simulink library "ddm"  (R2021b)
settings: Solver=VariableStepAuto  StartTime=0.0  StopTime=10.0  RelTol=1e-3
undefined symbols (not defined in the file or in its folder): ENUM_ADASACCSTA_ERROR, ENUM_ADASACCSTA_OFF, ENUM_ADASACCSTA_STANDBY, ENUM_ADASISASTA_OFF, ENUM_ALLOWMOV_ALLOWREADY, ENUM_APS, ENUM_BRKSTA_ERROR, ENUM_BRKSTA_OFF, ENUM_BRKSTA_ON, ENUM_BRKSW_INVALID, ENUM_BRKSW_OFF, ENUM_BRKSW_ON, ENUM_CHGPREACTERRSTA_OBCPRE, ENUM_DCDCFAULTSTA_ANYFAULTLV1, ENUM_DCDCFAULTSTA_ANYFAULTLV2, ENUM_DRIVETRAIN_AWD, ENUM_DRIVETRAIN_FWD, ENUM_DRIVETRAIN_RWD, ENUM_DRSEATSTA_INVALID, ENUM_EDUDRTSTA_NORMAL, ENUM_EPBSTA_APPLIED, ENUM_EPBSTA_RELEASED, ENUM_HVBATTREADYPRE_READY, ENUM_MCUWARN_LV0, ENUM_MCUWARN_LV1, ENUM_MCUWARN_LV2, ENUM_MCUWARN_LV3, ENUM_MCUWARN_NOERROR, ENUM_OBCFAULTSTA_ANYFAULT, ENUM_PAS_R2F2, ENUM_PDFAULT_BATTPDFAIL, ENUM_PDFAULT_DCDCDISABLE, ENUM_PDFAULT_MCUDISABLE, ENUM_PDFAULT_MCUDISCHRG, ENUM_POWERSTA_OFF, ENUM_POWERSTA_ON, ENUM_POWERSTA_READY, ENUM_POWERSTA_STANDBY, ENUM_PRESSINDI_LOW, ENUM_PUFAULT_BATTUPFAIL, ENUM_PUFAULT_DCDCENABLEFAIL, ENUM_PUFAULT_PRECHRGCHKFAIL, ENUM_PUFAULT_SAFETYCHKFAIL, ENUM_PUSTATE_COMPLETED, ENUM_PWRSTASW_OFF, ENUM_PWRSTASW_OFFA, ENUM_PWRSTASW_OFFCHVCHRG, ENUM_PWRSTASW_OFFCLVCHRG, ENUM_PWRSTASW_ON, ENUM_PWRSTASW_ONHVCHRG, ENUM_PWRSTASW_READY, ENUM_PWRSTASW_STANDBY, ENUM_RANGESTA_12IN, ENUM_SHIFTCOMMAND_D, ENUM_SHIFTCOMMAND_N, ENUM_SHIFTCOMMAND_P, ENUM_SHIFTCOMMAND_R, ENUM_VEHMALFUNLV_2ND, ENUM_VEHMALFUNLV_3RD, ENUM_VEHMALFUNLV_4TH ... (+835)
libraries: hcu_lib x750, $bdroot x12, simulink x5
(part 15 of 28)

== system ddm/DDM/DDM/PMM/Brake switch signal abnormal/Brake switch signal abnormal and no backup signal ==
  note: Diagnostics and Fault Handling
  note: Release Condition During Failure Detection
  note: Test Detection Criteria
  note: Release Condition After Failure Decision
  note: Fail Safe Operation During Failure Detection
  note: Test Pass Criteria
  note: Fail Safe Operation After Failure Decision
  task_time_s : Inport
  VPMM_PowerSta_enum : Inport  Port=2
  VPMM_PwrStaSW_enum : Inport  Port=3
  BrkSWNoBac : Inport  Port=4
  BrkSWPass : Inport  Port=5
  DTC_clear_request : Inport  Port=6
  VDDM_BrakeSW_enum : Inport  Port=7
  Constant1 : Constant  Value=ENUM_PWRSTASW_READY
  Constant11 : Constant  Value=KDDM_BrkSWNoBacPassSW_flg
  Constant15 : Constant  Value=KDDM_BrkSWNoBacCFSSW_flg
  Constant19 : Constant  Value=ENUM_POWERSTA_OFF
  Constant2 : Constant  Value=ENUM_PWRSTASW_ON
  Constant20 : Constant  Value=KDDM_BrkSWNoBacDFSSW_flg
  Constant23 : Constant  Value=TRUE
  Constant24 : Constant  Value=TRUE
  Constant25 : Constant  Value=FALSE
  Constant26 : Constant  Value=ENUM_PWRSTASW_READY
  Constant27 : Constant  Value=FALSE
  Constant28 : Constant  Value=ENUM_PWRSTASW_ON
  Constant29 : Constant  Value=ENUM_PWRSTASW_ONHVCHRG
  Constant3 : Constant  Value=ENUM_PWRSTASW_ONHVCHRG
  Constant38 : Constant  Value=KDDM_BrkSWNoBacDetTO_s
  Constant4 : Constant  Value=KDDM_BrkSWNoBacPassTO_s
  Constant40 : Constant  Value=KDDM_BrkSWNoBacDTC_cnt
  Constant42 : Constant  Value=ENUM_DRSEATSTA_INVALID
  Constant43 : Constant  Value=KDDM_BrkSWNoBacPassTO_s
  Constant44 : Constant  Value=KDDM_BrkSWNoBacDetSW_flg
  Constant5 : Constant  Value=KDDM_BrkSWNoBacDTC_cnt
  Constant8 : Constant  Value=FALSE
  DTC_Couter : hcu_lib/Basic_Blocks/DTC_Couter
  DTC_Info : hcu_lib/Basic_Blocks/DTC_Info
  Data Type Conversion1 : DataTypeConversion  OutDataTypeStr=uint8
  Equal{1..2,4..8} (7 alike) : RelationalOperator  Operator===  OutDataTypeStr=boolean  RndMeth=Simplest
  Equal3 : RelationalOperator  OutDataTypeStr=boolean  RndMeth=Simplest
  Logical Operator1 : Logic  Operator=NOT  AllPortsSameDT=off  OutDataTypeStr=boolean
  Logical Operator12 : Logic  AllPortsSameDT=off  OutDataTypeStr=boolean
  Logical Operator15 : Logic  AllPortsSameDT=off  OutDataTypeStr=boolean
  Logical Operator18 : Logic  AllPortsSameDT=off  OutDataTypeStr=boolean
  Logical Operator19 : Logic  Inputs=3  AllPortsSameDT=off  OutDataTypeStr=boolean
  Logical Operator2 : Logic  Operator=OR  Inputs=3  AllPortsSameDT=off  OutDataTypeStr=boolean
  Logical Operator3 : Logic  Operator=OR  Inputs=3  AllPortsSameDT=off  OutDataTypeStr=boolean
  Logical Operator4 : Logic  Operator=OR  AllPortsSameDT=off  OutDataTypeStr=boolean
  Logical Operator5 : Logic  Operator=OR  Inputs=3  AllPortsSameDT=off  OutDataTypeStr=boolean
  Logical Operator6 : Logic  Operator=NOT  AllPortsSameDT=off  OutDataTypeStr=boolean
  Logical Operator7 : Logic  Operator=OR  AllPortsSameDT=off  OutDataTypeStr=boolean
  Logical Operator8 : Logic  Operator=OR  AllPortsSameDT=off  OutDataTypeStr=boolean
  Relay : Relay  OnSwitchValue=ONE_INT  OffSwitchValue=ZERO_INT
  SR_Latch1 : Subsystem  mask(SR_Latch){}
      mask help: SR latch function.
  SR_Latch3 : hcu_lib/Basic_Blocks/SR_Latch
  SR_Latch4 : hcu_lib/Basic_Blocks/SR_Latch
  Switch{,2,4..6} (5 alike) : Switch  Criteria=u2 ~= 0
  Test Detection Criteria : hcu_lib/Basic_Blocks/Test Detection Criteria
  Timer1 : hcu_lib/Basic_Blocks/Timer
  VDDM_BrkSWNoBacDTC_raw32 : Outport
  VDDM_VCUBrkSWSta_enum : Outport  Port=2
  wires:
  Relay/1 -> SR_Latch3/1
  Data Type Conversion1/1 -> [VDDM_BrkSWNoBacDTC_cnt]  "VDDM_BrkSWNoBacDTC_cnt"
  Logical Operator19/1 -> DTC_Couter/1
  DTC_Couter/1 -> SR_Latch4/1
  Constant15/1 -> Logical Operator18/2
  [VDDM_BrkSWNoBacCFS_flg] -> Logical Operator7/1
  Constant44/1 -> Logical Operator19/2
  Logical Operator4/1 -> SR_Latch4/2
  SR_Latch3/1 -> Logical Operator12/2
  [VDDM_BrkSWNoBacCFSRls_flg] -> Logical Operator3/2
  [DTC_clear_request] -> Logical Operator1/1
  Logical Operator1/1 -> Logical Operator19/3
  [VDDM_BrkSWNoBacDTC_cnt] -> Relay/1
  DTC_Couter/2 -> Data Type Conversion1/1
  Logical Operator18/1 -> [VDDM_BrkSWNoBacCFS_flg]  "VDDM_BrkSWNoBacCFS_flg"
  Constant11/1 -> Logical Operator15/2
  [VDDM_BrkSWNoBacDet_flg] -> Logical Operator19/1
  Constant20/1 -> Logical Operator12/1
  Logical Operator7/1 -> SR_Latch3/2
  [VDDM_BrkSWNoBacPass_flg] -> Logical Operator3/1
  Constant5/1 -> DTC_Couter/3
  SR_Latch4/1 -> Logical Operator18/1
  Logical Operator3/1 -> Logical Operator15/1
  [VDDM_BrkSWNoBacCFSRls_flg] -> Logical Operator4/1
  Logical Operator12/1 -> [VDDM_BrkSWNoBacDFS_flg]  "VDDM_BrkSWNoBacDFS_flg"
  Logical Operator15/1 -> DTC_Couter/2
  [DTC_clear_request] -> Logical Operator4/2
  [DTC_clear_request] -> Logical Operator7/2
  [DTC_clear_request] -> Logical Operator3/3
  VDDM_BrakeSW_enum/1 -> [VDDM_BrakeSW_enum]
  Constant8/1 -> Switch6/1
  Switch5/1 -> Switch6/3
  Switch6/1 -> Test Detection Criteria/1
  [DTC_clear_request] -> Switch6/2
  [DTC_clear_request] -> DTC_Info/4
  Constant38/1 -> Test Detection Criteria/4
  [VDDM_BrkSWNoBacDet_flg] -> DTC_Info/1
  BrkSWPass/1 -> Switch2/1
  BrkSWNoBac/1 -> Switch5/1
  [VDDM_BrkSWNoBacCFS_flg] -> DTC_Info/3
  [VDDM_BrkSWNoBacPass_flg] -> DTC_Info/2
  DTC_Info/1 -> VDDM_BrkSWNoBacDTC_raw32/1  "VDDM_BrkSWNoBacDTC_raw32"
  [task_time_s] -> Timer1/3
  DTC_clear_request/1 -> [DTC_clear_request]
  [VDDM_VCUBrkSWSta_enum] -> VDDM_VCUBrkSWSta_enum/1
  Constant26/1 -> Equal1/2
  [VPMM_PwrStaSW_enum] -> Equal1/1
  Constant40/1 -> Test Detection Criteria/3
  [VPMM_PwrStaSW_enum] -> Equal5/1
  [VPMM_PwrStaSW_enum] -> Equal6/1
  Logical Operator2/1 -> Switch5/2
  Switch/1 -> [VDDM_VCUBrkSWSta_enum]  "VDDM_VCUBrkSWSta_enum"
  SR_Latch1/1(latched) -> [VDDM_BrkSWNoBacPass_flg]  "VDDM_BrkSWNoBacPass_flg"
  [VPMM_PowerSta_enum] -> Equal4/1
  Constant24/1 -> Switch4/1
  Constant42/1 -> Switch/1
  Switch2/1 -> Timer1/1, Logical Operator6/1, SR_Latch1/2(reset)
  Equal3/1 -> SR_Latch1/1(set)
  Switch4/1 -> [VDDM_BrkSWNoBacCFSRls_flg]  "VDDM_BrkSWNoBacCFSRls_flg"
  Constant19/1 -> Equal4/2
  Constant25/1 -> Switch4/3
  [DTC_clear_request] -> Logical Operator8/2
  Logical Operator8/1 -> Switch4/2
  Equal4/1 -> Logical Operator8/1
  Constant27/1 -> Switch5/3
  Constant23/1 -> Switch2/3
  [VDDM_BrkSWNoBacCFS_flg] -> Switch/2
  [VDDM_BrakeSW_enum] -> Switch/3
  Test Detection Criteria/1 -> [VDDM_BrkSWNoBacDet_flg]  "VDDM_BrkSWNoBacDet_flg"
  [task_time_s] -> Test Detection Criteria/2
  Timer1/1 -> Equal3/1
  Constant43/1 -> Timer1/4
  Constant29/1 -> Equal6/2
  Constant4/1 -> Equal3/2
  Constant28/1 -> Equal5/2
  VPMM_PowerSta_enum/1 -> [VPMM_PowerSta_enum]
  VPMM_PwrStaSW_enum/1 -> [VPMM_PwrStaSW_enum]
  task_time_s/1 -> [task_time_s]
  Logical Operator6/1 -> Timer1/2
  Equal5/1 -> Logical Operator2/1
  Equal1/1 -> Logical Operator2/2
  Equal6/1 -> Logical Operator2/3
  [VPMM_PwrStaSW_enum] -> Equal2/1
  Constant2/1 -> Equal7/2
  [VPMM_PwrStaSW_enum] -> Equal8/1
  Equal2/1 -> Logical Operator5/2
  Equal7/1 -> Logical Operator5/1
  Equal8/1 -> Logical Operator5/3
  Logical Operator5/1 -> Switch2/2
  [VPMM_PwrStaSW_enum] -> Equal7/1
  Constant3/1 -> Equal8/2
  Constant1/1 -> Equal2/2

== system ddm/DDM/DDM/PMM/Brake switch signal abnormal/Subsystem ==
  note: 17
  note: 6
  note: 35
  note: 25
  note: 27
  note: 30
  note: 12
  note: 19
  note: 3
  note: 21
  note: 1
  note: 9
  note: 11
  note: 36
  note: 24
  note: 33
  note: 29
  note: 13
  note: 5
  note: 23
  note: 18
  note: 15
  VDDM_CANBSW2S_enum : Inport
  BrakeSW : Inport  Port=2
  Brake_Stop_Lamp : Inport  Port=3
  BrkPedalPos_enum : Inport  Port=4
  1-D Lookup Table : Lookup_n-D  NumberOfTableDimensions=1  BreakpointsForDimension1=[1:36]  Table=[20,8,32,18,6,30,19,7,31,16,4,28,17,5,29,15,3,27,14,2,26,13,1,25,24,12,36,23,11,35,22,10,34,21,9,33]  ExtrapMethod=Clip  InternalRulePriority=Speed  RndMeth=Simplest  InputSameDT=on
  AND{,2..7,10,12..25} (22 alike) : Logic  Inputs=4  AllPortsSameDT=off  OutDataTypeStr=boolean
  AND1 : Logic  Operator=OR  Inputs=6  AllPortsSameDT=off  OutDataTypeStr=boolean
  AND11 : Logic  Operator=OR  Inputs=15  AllPortsSameDT=off  OutDataTypeStr=boolean
  AND8 : Logic  Operator=OR  AllPortsSameDT=off  OutDataTypeStr=boolean
  AND9 : Logic  Operator=OR  AllPortsSameDT=off  OutDataTypeStr=boolean
  Constant{1..10,15,17..18,23,29..30,32} (17 alike) : Constant  Value=ENUM_BRKSTA_ON
  Constant11 : Constant  Value=ENUM_BRKSW_OFF
  Constant{16,19,21,25..28,31,38,50,53,55,57,59..61} (16 alike) : Constant  Value=ENUM_BRKSTA_ERROR
  Constant{20,22,24,33..34,39,41..44} (10 alike) : Constant  Value=ENUM_BRKSTA_OFF
  Constant35 : Constant  Value=FALSE
  Constant36 : Constant  Value=TRUE
  Constant37 : Constant  Value=0
  Constant40 : Constant  Value=0
  Constant46 : Constant  Value=ENUM_BRKSW_ON
  Constant47 : Constant  Value=ENUM_BRKSW_INVALID
  Data Type Conversion{,1..3} (4 alike) : DataTypeConversion
  Equal{1..45} (45 alike) : RelationalOperator  Operator===  OutDataTypeStr=boolean  RndMeth=Simplest
  OR{,1..21} (22 alike) : Logic  Operator=NOT  AllPortsSameDT=off  OutDataTypeStr=boolean
  Switch6 : Switch  Criteria=u2 > Threshold
  Switch7 : Switch  Criteria=u2 > Threshold
  Switch8 : Switch  Criteria=u2 > Threshold
  n-D Lookup Table : Lookup_n-D  NumberOfTableDimensions=4  BreakpointsForDimension1=[0:2]  BreakpointsForDimension2=[0:1]  BreakpointsForDimension3=[0:1]  BreakpointsForDimension4=[0:2]  Table=reshape(1:36,[3,2,2,3])  ExtrapMethod=Clip  InternalRulePriority=Speed  RndMeth=Simplest  InputSameDT=on
      settings: InputPortMap=u0,u1,u2,u3
  BrkSWErr : Outport
  BrkSWNoBac : Outport  Port=2
  BrkSWPass : Outport  Port=3
  VDDM_BrakeSW_enum : Outport  Port=4
  wires:
  [VDDM_BrakeSW_enum] -> VDDM_BrakeSW_enum/1
  [BrkSWPass] -> BrkSWPass/1
  [BrkSWNoBac] -> BrkSWNoBac/1
  [BrkSWErr] -> BrkSWErr/1
  BrkPedalPos_enum/1 -> [BrkPedalPos_enum]
  Brake_Stop_Lamp/1 -> [Brake_Stop_Lamp]
  BrakeSW/1 -> [BrakeSW]
  VDDM_CANBSW2S_enum/1 -> [VDDM_CANBSW2S_enum]
  AND4/1 -> AND1/4
  Constant28/1 -> Equal14/2
  AND25/1 -> AND11/15
  Constant31/1 -> Equal13/2
  Equal22/1 -> AND10/3
  Constant7/1 -> Equal3/2
  Equal33/1 -> AND19/4
  Equal39/1 -> AND22/4
  OR1/1 -> AND2/3
  [Brake_Stop_Lamp] -> OR8/1
  [Brake_Stop_Lamp] -> OR10/1
  Constant8/1 -> Equal8/2
  Equal17/1 -> AND7/1
  Constant50/1 -> Equal35/2
  Constant32/1 -> Equal41/2
  [BrkPedalPos_enum] -> Equal35/1
  Equal43/1 -> AND24/4
  Constant33/1 -> Equal26/2
  [VDDM_CANBSW2S_enum] -> Equal9/1
  Constant37/1 -> Equal20/2
  [BrkPedalPos_enum] -> Equal45/1
  Switch7/1 -> Switch8/3
  Equal36/1 -> AND21/1
  [Brake_Stop_Lamp] -> AND5/3
  Constant3/1 -> Equal17/2
  Constant44/1 -> Equal43/2
  Constant39/1 -> Equal30/2
  OR8/1 -> AND13/3
  [Brake_Stop_Lamp] -> OR19/1
  [VDDM_CANBSW2S_enum] -> Equal20/1
  Equal20/1 -> AND10/1
  [Brake_Stop_Lamp] -> Equal22/1
  [BrkPedalPos_enum] -> Equal6/1
  [VDDM_CANBSW2S_enum] -> Equal2/1
  Equal5/1 -> AND3/1
  [Brake_Stop_Lamp] -> OR3/1
  [Brake_Stop_Lamp] -> OR15/1
  Constant26/1 -> Equal11/2
  [Brake_Stop_Lamp] -> AND21/3
  OR19/1 -> AND24/3
  [BrkPedalPos_enum] -> Equal10/1
  [BrakeSW] -> AND25/2
  OR3/1 -> AND4/3
  Equal31/1 -> AND18/4
  [BrkPedalPos_enum] -> Equal31/1
  [VDDM_CANBSW2S_enum] -> Equal38/1
  Equal13/1 -> AND6/4
  AND9/1 -> Switch6/2
  [VDDM_CANBSW2S_enum] -> Equal17/1
  AND14/1 -> AND11/4
  [Brake_Stop_Lamp] -> AND16/3
  Equal18/1 -> AND7/4
  [BrkPedalPos_enum] -> Equal27/1
  Constant61/1 -> Equal44/2
  Equal14/1 -> AND6/1
  [VDDM_CANBSW2S_enum] -> Equal5/1
  [VDDM_CANBSW2S_enum] -> Equal28/1
  [VDDM_CANBSW2S_enum] -> Equal3/1
  [BrkPedalPos_enum] -> Equal8/1
  [Brake_Stop_Lamp] -> OR14/1
  AND17/1 -> AND11/7
  Constant30/1 -> Equal16/2
  Constant43/1 -> Equal34/2
  OR13/1 -> AND18/2
  Equal26/1 -> AND16/1
  OR7/1 -> AND13/2
  [BrakeSW] -> AND24/2
  Equal16/1 -> AND/1
  Equal34/1 -> AND20/1
  Equal9/1 -> AND14/1
  Equal12/1 -> AND5/4
  [VDDM_CANBSW2S_enum] -> Equal24/1
  Constant16/1 -> Equal1/2
  Constant18/1 -> Equal31/2
  Constant9/1 -> Equal9/2
  AND2/1 -> AND1/2
  Constant40/1 -> Equal19/2
  OR17/1 -> AND23/2
  AND5/1 -> AND1/5
  AND6/1 -> AND1/6
  Equal37/1 -> AND21/4
  Constant25/1 -> Equal10/2
  [BrkPedalPos_enum] -> Equal15/1
  Constant21/1 -> Equal6/2
  [BrkPedalPos_enum] -> Equal29/1
  [VDDM_CANBSW2S_enum] -> Equal34/1
  [BrkPedalPos_enum] -> Equal23/1
  AND19/1 -> AND11/9
  Constant15/1 -> Equal27/2
  Equal27/1 -> AND16/4
  OR14/1 -> AND19/3
  [BrkPedalPos_enum] -> Equal43/1
  [VDDM_CANBSW2S_enum] -> Equal26/1
  [BrakeSW] -> AND16/2
  AND15/1 -> AND11/5
  Equal24/1 -> AND2/1
  Constant6/1 -> Equal23/2
  AND10/1 -> AND8/1
  OR11/1 -> AND17/3
  [BrakeSW] -> AND14/2
  [BrakeSW] -> AND17/2
  Constant38/1 -> Equal21/2
  [BrkPedalPos_enum] -> Equal41/1
  [BrakeSW] -> AND3/2
  Equal7/1 -> AND4/1
  Equal28/1 -> AND17/1
  OR16/1 -> AND22/3
  AND13/1 -> AND11/3
  Equal23/1 -> AND12/4
  Equal25/1 -> AND15/1
  Constant57/1 -> Equal40/2
  [VDDM_CANBSW2S_enum] -> Equal11/1
  Constant55/1 -> Equal38/2
  OR6/1 -> AND10/2
  AND16/1 -> AND11/6
  Equal10/1 -> AND4/4
  OR9/1 -> AND14/3
  AND8/1 -> AND9/2, [BrkSWPass]
  Constant1/1 -> Equal24/2
  [BrakeSW] -> AND20/2
  Equal19/1 -> AND10/4
  Constant36/1 -> Switch6/3
  [VDDM_CANBSW2S_enum] -> Equal40/1
  [BrakeSW] -> AND19/2
  [BrkPedalPos_enum] -> Equal1/1
  AND12/1 -> AND11/2
  Constant4/1 -> Equal18/2
  [VDDM_CANBSW2S_enum] -> Equal14/1
  [Brake_Stop_Lamp] -> AND/3
  [BrkPedalPos_enum] -> Equal37/1
  Constant60/1 -> Equal45/2
  Constant5/1 -> Equal2/2
  Constant20/1 -> Equal5/2
  [BrakeSW] -> AND22/2
  [BrakeSW] -> AND21/2
  Constant53/1 -> Equal36/2
  Equal35/1 -> AND20/4
  [VDDM_CANBSW2S_enum] -> Equal16/1
  [BrakeSW] -> OR7/1
  Constant10/1 -> Equal25/2
  [Brake_Stop_Lamp] -> OR5/1
  [Brake_Stop_Lamp] -> AND3/3
  Equal6/1 -> AND3/4
  Constant42/1 -> Equal33/2
  AND22/1 -> AND11/12
  AND7/1 -> AND8/2, AND11/1
  [VDDM_CANBSW2S_enum] -> Equal30/1
  [BrakeSW] -> OR/1
  Equal41/1 -> AND23/4
  OR12/1 -> AND18/3
  [Brake_Stop_Lamp] -> OR12/1
  [VDDM_CANBSW2S_enum] -> Equal36/1
  Constant24/1 -> Equal15/2
  [Brake_Stop_Lamp] -> OR16/1
  Constant41/1 -> Equal32/2
  Equal32/1 -> AND19/1
  Switch8/1 -> [VDDM_BrakeSW_enum]
  Constant17/1 -> Equal29/2
  Equal45/1 -> AND25/4
  Constant19/1 -> Equal4/2
  [BrakeSW] -> AND7/2
  OR21/1 -> AND7/3
  Constant47/1 -> Switch8/1
  [Brake_Stop_Lamp] -> OR21/1
  [Brake_Stop_Lamp] -> OR9/1
  Equal40/1 -> AND23/1
  Equal3/1 -> AND13/1
  Equal11/1 -> AND5/1
  Equal38/1 -> AND22/1
  Constant11/1 -> Switch7/3
  Equal1/1 -> AND/4
  Switch6/1 -> [BrkSWErr]
  [BrkPedalPos_enum] -> Equal13/1
  [BrkPedalPos_enum] -> Equal21/1
  AND24/1 -> AND11/14
  Constant35/1 -> Switch6/1
  AND/1 -> AND1/1
  Constant34/1 -> Equal28/2
  [VDDM_CANBSW2S_enum] -> Equal44/1
  OR10/1 -> AND15/3
  [Brake_Stop_Lamp] -> AND12/3
  [BrkPedalPos_enum] -> Equal18/1
  Equal8/1 -> AND13/4
  Equal2/1 -> AND12/1
  [BrkPedalPos_enum] -> Equal4/1
  [Brake_Stop_Lamp] -> OR11/1
  Equal44/1 -> AND25/1
  Equal42/1 -> AND24/1
  [BrakeSW] -> OR4/1
  OR20/1 -> AND25/3
  [VDDM_CANBSW2S_enum] -> Equal7/1
  OR4/1 -> AND6/2
  Constant23/1 -> Equal37/2
  [VDDM_CANBSW2S_enum] -> Equal32/1
  [VDDM_CANBSW2S_enum] -> Equal42/1
  [BrkPedalPos_enum] -> Equal19/1
  [BrkPedalPos_enum] -> Equal12/1
  AND21/1 -> AND11/11
  [BrkPedalPos_enum] -> Equal39/1
  [BrakeSW] -> OR6/1
  Constant59/1 -> Equal42/2
  AND1/1 -> [BrkSWNoBac], AND9/1, Switch8/2
  AND23/1 -> AND11/13
  Constant27/1 -> Equal12/2
  AND18/1 -> AND11/8
  AND20/1 -> AND11/10
  [BrakeSW] -> AND15/2
  Constant46/1 -> Switch7/1
  AND11/1 -> Switch7/2
  [BrakeSW] -> OR2/1
  [VDDM_CANBSW2S_enum] -> Equal25/1
  Constant2/1 -> Equal22/2
  [Brake_Stop_Lamp] -> OR1/1
  [Brake_Stop_Lamp] -> OR18/1
  [BrakeSW] -> OR13/1
  OR5/1 -> AND6/3
  Constant22/1 -> Equal7/2
  Constant29/1 -> Equal39/2
  OR18/1 -> AND23/3
  [BrakeSW] -> AND/2
  [BrakeSW] -> OR17/1
  AND3/1 -> AND1/3
  [BrakeSW] -> AND12/2
  [Brake_Stop_Lamp] -> OR20/1
  OR15/1 -> AND20/3
  OR/1 -> AND2/2
  Equal21/1 -> AND15/4
  Equal30/1 -> AND18/1
  Equal29/1 -> AND17/4
  Equal15/1 -> AND14/4
  [BrakeSW] -> AND5/2
  OR2/1 -> AND4/2
  Equal4/1 -> AND2/4
  [BrkPedalPos_enum] -> Equal33/1
  Data Type Conversion2/1 -> n-D Lookup Table/3
  Data Type Conversion3/1 -> n-D Lookup Table/4
  Data Type Conversion1/1 -> n-D Lookup Table/2
  Data Type Conversion/1 -> n-D Lookup Table/1
  [BrakeSW] -> Data Type Conversion1/1
  [BrkPedalPos_enum] -> Data Type Conversion3/1
  n-D Lookup Table/1 -> 1-D Lookup Table/1
  [Brake_Stop_Lamp] -> Data Type Conversion2/1
  1-D Lookup Table/1 -> [VDDM_BrakeSigMatrix_enum]  "VDDM_BrakeSigMatrix_enum"
  [VDDM_CANBSW2S_enum] -> Data Type Conversion/1

== system ddm/DDM/DDM/PMM/Comm err/FDC lost communication with EPAS2 ==
  note: Diagnostics and Fault Handling
  note: Release Condition During Failure Detection
  note: Release Condition After Failure Decision
  note: Fail Safe During Detection
  note: Test Detection Criteria
  note: Test Pass Criteria
  note: Fail Safe After Decision
  task_time_s : Inport
  VPMM_PowerSta_enum : Inport  Port=2
  VPMM_PwrStaSW_enum : Inport  Port=3
  VDDM_C1EPAS2LCChk_flg : Inport  Port=4
  No_CAN1_BUS_OFF : Inport  Port=5
  DTC_clear_request : Inport  Port=6
  Constant15 : Constant  Value=KDDM_C1EPAS2LCCFSSW_flg
  Constant16 : Constant  Value=TRUE
  Constant18 : Constant  Value=KDDM_C1EPAS2LCPassTO_s
  Constant19 : Constant  Value=KDDM_C1EPAS2LCPassTO_s
  Constant{2,21,25,27} (4 alike) : Constant  Value=FALSE
  Constant20 : Constant  Value=KDDM_C1EPAS2LCDFSSW_flg
  Constant24 : Constant  Value=TRUE
  Constant26 : Constant  Value=ENUM_PWRSTASW_OFF
  Constant28 : Constant  Value=ENUM_PWRSTASW_OFF
  Constant3 : Constant  Value=TRUE
  Constant4 : Constant  Value=ENUM_POWERSTA_OFF
  Constant40 : Constant  Value=KDDM_C1EPAS2LCDTC_cnt
  Constant41 : Constant  Value=KDDM_C1EPAS2LCDetTO_s
  Constant46 : Constant  Value=KDDM_C1EPAS2LCDetSW_flg
  Constant48 : Constant  Value=KDDM_C1EPAS2LCDTC_cnt
  Constant5 : Constant  Value=KDDM_C1EPAS2LCPassSW_flg
  DTC_Couter : hcu_lib/Basic_Blocks/DTC_Couter
  DTC_Info : hcu_lib/Basic_Blocks/DTC_Info
  Data Type Conversion1 : DataTypeConversion  OutDataTypeStr=uint8
  Equal : RelationalOperator  Operator=~=  OutDataTypeStr=boolean  RndMeth=Simplest
  Equal2 : RelationalOperator  Operator=~=  OutDataTypeStr=boolean  RndMeth=Simplest
  Equal3 : RelationalOperator  OutDataTypeStr=boolean  RndMeth=Simplest
  Equal4 : RelationalOperator  Operator===  OutDataTypeStr=boolean  RndMeth=Simplest
  Goto19 : Goto  Commented=on  GotoTag=EDriveSysErr_VCUErr_flg
  Logical Operator1 : Logic  Operator=NOT  AllPortsSameDT=off  OutDataTypeStr=boolean
  Logical Operator{2,5,12,15,18} (5 alike) : Logic  AllPortsSameDT=off  OutDataTypeStr=boolean
  Logical Operator19 : Logic  Inputs=3  AllPortsSameDT=off  OutDataTypeStr=boolean
  Logical Operator3 : Logic  Operator=OR  Inputs=3  AllPortsSameDT=off  OutDataTypeStr=boolean
  Logical Operator4 : Logic  Operator=OR  AllPortsSameDT=off  OutDataTypeStr=boolean
  Logical Operator6 : Logic  Operator=NOT  AllPortsSameDT=off  OutDataTypeStr=boolean
  Logical Operator7 : Logic  Operator=OR  AllPortsSameDT=off  OutDataTypeStr=boolean
  Logical Operator8 : Logic  Operator=OR  AllPortsSameDT=off  OutDataTypeStr=boolean
  Relay : Relay  OnSwitchValue=ONE_INT  OffSwitchValue=ZERO_INT
  SR_Latch1 : Subsystem  mask(SR_Latch){}
      mask help: SR latch function.
  SR_Latch3 : hcu_lib/Basic_Blocks/SR_Latch
  SR_Latch4 : hcu_lib/Basic_Blocks/SR_Latch
  Switch{,1,4..6} (5 alike) : Switch  Criteria=u2 ~= 0
  Test Detection Criteria : hcu_lib/Basic_Blocks/Test Detection Criteria
  Timer1 : hcu_lib/Basic_Blocks/Timer
  VDDM_C1EPAS2LCDTC_raw32 : Outport
  VDDM_C1EPAS2LCCFS_flg : Outport  Port=2
  wires:
  [DTC_clear_request] -> Logical Operator1/1
  Logical Operator3/1 -> Logical Operator15/1
  Constant46/1 -> Logical Operator19/2
  SR_Latch4/1 -> Logical Operator18/1
  [DTC_clear_request] -> Logical Operator7/2
  [VDDM_C1EPAS2LCCFS_flg] -> Logical Operator7/1
  DTC_Couter/1 -> SR_Latch4/1
  Logical Operator7/1 -> SR_Latch3/2
  Logical Operator4/1 -> SR_Latch4/2
  Constant48/1 -> DTC_Couter/3
  [VDDM_C1EPAS2LCDet_flg] -> Logical Operator19/1
  SR_Latch3/1 -> Logical Operator12/2
  Logical Operator15/1 -> DTC_Couter/2
  Logical Operator19/1 -> DTC_Couter/1
  [VDDM_C1EPAS2LCDTC_cnt] -> Relay/1
  Constant20/1 -> Logical Operator12/1
  DTC_Couter/2 -> Data Type Conversion1/1
  [DTC_clear_request] -> Logical Operator3/3
  Logical Operator1/1 -> Logical Operator19/3
  [VDDM_C1EPAS2LCCFSRls_flg] -> Logical Operator4/1
  Relay/1 -> SR_Latch3/1
  [VDDM_C1EPAS2LCCFSRls_flg] -> Logical Operator3/2
  Data Type Conversion1/1 -> [VDDM_C1EPAS2LCDTC_cnt]  "VDDM_C1EPAS2LCDTC_cnt"
  Logical Operator12/1 -> [VDDM_C1EPAS2LCDFS_flg]  "VDDM_C1EPAS2LCDFS_flg"
  Constant15/1 -> Logical Operator18/2
  [DTC_clear_request] -> Logical Operator4/2
  Logical Operator18/1 -> [VDDM_C1EPAS2LCCFS_flg]  "VDDM_C1EPAS2LCCFS_flg"
  Constant5/1 -> Logical Operator15/2
  [VDDM_C1EPAS2LCPass_flg] -> Logical Operator3/1
  Test Detection Criteria/1 -> [VDDM_C1EPAS2LCDet_flg]  "VDDM_C1EPAS2LCDet_flg"
  VPMM_PowerSta_enum/1 -> [VPMM_PowerSta_enum]
  VPMM_PwrStaSW_enum/1 -> [VPMM_PwrStaSW_enum]
  VDDM_C1EPAS2LCChk_flg/1 -> [VDDM_C1EPAS2LCChk_flg]
  task_time_s/1 -> [task_time_s]
  DTC_clear_request/1 -> [DTC_clear_request]
  No_CAN1_BUS_OFF/1 -> [No_CAN1_BUS_OFF]
  Constant3/1 -> Switch/1
  Constant19/1 -> Equal3/2
  Constant16/1 -> Switch6/3
  Logical Operator6/1 -> Timer1/1
  [task_time_s] -> Test Detection Criteria/2
  Equal/1 -> Logical Operator2/2
  Equal4/1 -> Logical Operator8/1
  Timer1/1 -> Equal3/1
  Constant27/1 -> Switch5/3
  [No_CAN1_BUS_OFF] -> Logical Operator2/1
  [DTC_clear_request] -> Logical Operator8/2
  Constant26/1 -> Equal/2
  Constant24/1 -> Switch4/1
  Logical Operator2/1 -> Switch5/2
  Logical Operator5/1 -> Switch6/2
  Switch/1 -> Goto19/1
  [No_CAN1_BUS_OFF] -> Logical Operator5/1
  [VDDM_xxx_flg] -> SR_Latch1/2(reset)
  Constant40/1 -> Test Detection Criteria/3
  Constant21/1 -> Switch/3
  [VDDM_C1EPAS2LCCFS_flg] -> Switch/2
  Equal2/1 -> Logical Operator5/2
  Constant25/1 -> Switch4/3
  Switch4/1 -> [VDDM_C1EPAS2LCCFSRls_flg]  "VDDM_C1EPAS2LCCFSRls_flg"
  [VDDM_C1EPAS2LCChk_flg] -> Switch6/1
  Logical Operator8/1 -> Switch4/2
  [VDDM_C1EPAS2LCChk_flg] -> Switch5/1
  Constant28/1 -> Equal2/2
  SR_Latch1/1(latched) -> [VDDM_C1EPAS2LCPass_flg]  "VDDM_C1EPAS2LCPass_flg"
  Switch6/1 -> Logical Operator6/1, Timer1/2
  Equal3/1 -> SR_Latch1/1(set)
  Constant18/1 -> Timer1/4
  Constant4/1 -> Equal4/2
  [VPMM_PowerSta_enum] -> Equal4/1
  [VPMM_PwrStaSW_enum] -> Equal/1
  [VPMM_PwrStaSW_enum] -> Equal2/1
  [task_time_s] -> Timer1/3
  DTC_Info/1 -> VDDM_C1EPAS2LCDTC_raw32/1  "VDDM_C1EPAS2LCDTC_raw32"
  [VDDM_C1EPAS2LCCFS_flg] -> DTC_Info/3, VDDM_C1EPAS2LCCFS_flg/1
  [VDDM_C1EPAS2LCDet_flg] -> DTC_Info/1
  [VDDM_C1EPAS2LCPass_flg] -> DTC_Info/2
  Constant41/1 -> Test Detection Criteria/4
  [DTC_clear_request] -> DTC_Info/4
  [DTC_clear_request] -> Switch1/2
  Switch1/1 -> Test Detection Criteria/1
  Switch5/1 -> [VDDM_xxx_flg], Switch1/3
  Constant2/1 -> Switch1/1

== system ddm/DDM/DDM/PMM/Comm err/The CAN signal between VCU and ABM1 is discontinuous ==
  note: Diagnostics and Fault Handling
  note: Release Condition After Failure Decision
  note: Fail Safe After Decision
  note: Release Condition During Failure Detection
  note: Test Detection Criteria
  note: Test Pass Criteria
  note: Fail Safe During Detection
  task_time_s : Inport
  VPMM_PowerSta_enum : Inport  Port=2
  VPMM_PwrStaSW_enum : Inport  Port=3
  VDDM_C1ABM1RCChk_flg : Inport  Port=4
  VDDM_C1ABM1LCCFS_flg : Inport  Port=5
  No_CAN1_BUS_OFF : Inport  Port=6
  DTC_clear_request : Inport  Port=7
  Constant15 : Constant  Value=KDDM_C1ABM1RCCFSSW_flg
  Constant16 : Constant  Value=TRUE
  Constant18 : Constant  Value=KDDM_C1ABM1RCPassTO_s
  Constant19 : Constant  Value=KDDM_C1ABM1RCPassTO_s
  Constant{2,21,25,27} (4 alike) : Constant  Value=FALSE
  Constant20 : Constant  Value=KDDM_C1ABM1RCDFSSW_flg
  Constant24 : Constant  Value=TRUE
  Constant26 : Constant  Value=ENUM_PWRSTASW_OFF
  Constant28 : Constant  Value=ENUM_PWRSTASW_OFF
  Constant3 : Constant  Value=TRUE
  Constant4 : Constant  Value=ENUM_POWERSTA_OFF
  Constant40 : Constant  Value=KDDM_C1ABM1RCDTC_cnt
  Constant41 : Constant  Value=KDDM_C1ABM1RCDetTO_s
  Constant46 : Constant  Value=KDDM_C1ABM1RCDetSW_flg
  Constant48 : Constant  Value=KDDM_C1ABM1RCDTC_cnt
  Constant5 : Constant  Value=KDDM_C1ABM1RCPassSW_flg
  DTC_Couter : hcu_lib/Basic_Blocks/DTC_Couter
  DTC_Info : hcu_lib/Basic_Blocks/DTC_Info
  Data Type Conversion1 : DataTypeConversion  OutDataTypeStr=uint8
  Equal : RelationalOperator  Operator=~=  OutDataTypeStr=boolean  RndMeth=Simplest
  Equal2 : RelationalOperator  Operator=~=  OutDataTypeStr=boolean  RndMeth=Simplest
  Equal3 : RelationalOperator  OutDataTypeStr=boolean  RndMeth=Simplest
  Equal4 : RelationalOperator  Operator===  OutDataTypeStr=boolean  RndMeth=Simplest
  Logical Operator{1,4,6..7} (4 alike) : Logic  Operator=NOT  AllPortsSameDT=off  OutDataTypeStr=boolean
  Logical Operator10 : Logic  Operator=OR  AllPortsSameDT=off  OutDataTypeStr=boolean
  Logical Operator12 : Logic  AllPortsSameDT=off  OutDataTypeStr=boolean
  Logical Operator15 : Logic  AllPortsSameDT=off  OutDataTypeStr=boolean
  Logical Operator18 : Logic  AllPortsSameDT=off  OutDataTypeStr=boolean
  Logical Operator19 : Logic  Inputs=3  AllPortsSameDT=off  OutDataTypeStr=boolean
  Logical Operator2 : Logic  Inputs=3  AllPortsSameDT=off  OutDataTypeStr=boolean
  Logical Operator3 : Logic  Operator=OR  Inputs=3  AllPortsSameDT=off  OutDataTypeStr=boolean
  Logical Operator5 : Logic  Inputs=3  AllPortsSameDT=off  OutDataTypeStr=boolean
  Logical Operator8 : Logic  Operator=OR  AllPortsSameDT=off  OutDataTypeStr=boolean
  Logical Operator9 : Logic  Operator=OR  AllPortsSameDT=off  OutDataTypeStr=boolean
  Relay : Relay  OnSwitchValue=ONE_INT  OffSwitchValue=ZERO_INT
  SR_Latch1 : Subsystem  mask(SR_Latch){}
      mask help: SR latch function.
  SR_Latch3 : hcu_lib/Basic_Blocks/SR_Latch
  SR_Latch4 : hcu_lib/Basic_Blocks/SR_Latch
  Switch{,1,4..6} (5 alike) : Switch  Criteria=u2 ~= 0
  Test Detection Criteria : hcu_lib/Basic_Blocks/Test Detection Criteria
  Timer1 : hcu_lib/Basic_Blocks/Timer
  VDDM_C1ABM1RCDTC_raw32 : Outport
  RC_EDriveSysErr_VCUErr_flg : Outport  Port=2
  wires:
  Logical Operator19/1 -> DTC_Couter/1
  Logical Operator15/1 -> DTC_Couter/2
  Logical Operator3/1 -> Logical Operator15/1
  [VDDM_C1ABM1RCCFSRls_flg] -> Logical Operator9/1
  Logical Operator12/1 -> [VDDM_C1ABM1RCDFS_flg]  "VDDM_C1ABM1RCDFS_flg"
  Relay/1 -> SR_Latch3/1
  [VDDM_C1ABM1RCDet_flg] -> Logical Operator19/1
  [DTC_clear_request] -> Logical Operator3/3
  [DTC_clear_request] -> Logical Operator7/1
  Data Type Conversion1/1 -> [VDDM_C1ABM1RCDTC_cnt]  "VDDM_C1ABM1RCDTC_cnt"
  [VDDM_C1ABM1RCDTC_cnt] -> Relay/1
  SR_Latch3/1 -> Logical Operator12/2
  [VDDM_C1ABM1RCCFS_flg] -> Logical Operator10/1
  Constant48/1 -> DTC_Couter/3
  Constant46/1 -> Logical Operator19/2
  Logical Operator7/1 -> Logical Operator19/3
  Constant20/1 -> Logical Operator12/1
  SR_Latch4/1 -> Logical Operator18/1
  [DTC_clear_request] -> Logical Operator9/2
  Constant5/1 -> Logical Operator15/2
  [DTC_clear_request] -> Logical Operator10/2
  Logical Operator10/1 -> SR_Latch3/2
  Logical Operator9/1 -> SR_Latch4/2
  [VDDM_C1ABM1RCPass_flg] -> Logical Operator3/1
  DTC_Couter/2 -> Data Type Conversion1/1
  DTC_Couter/1 -> SR_Latch4/1
  Logical Operator18/1 -> [VDDM_C1ABM1RCCFS_flg]  "VDDM_C1ABM1RCCFS_flg"
  [VDDM_C1ABM1RCCFSRls_flg] -> Logical Operator3/2
  Constant15/1 -> Logical Operator18/2
  Constant2/1 -> Switch1/1
  Switch5/1 -> Switch1/3, [VDDM_xxx_flg]
  Switch1/1 -> Test Detection Criteria/1
  [DTC_clear_request] -> Switch1/2
  [DTC_clear_request] -> DTC_Info/4
  Constant41/1 -> Test Detection Criteria/4
  [VDDM_C1ABM1RCDet_flg] -> DTC_Info/1
  [VDDM_C1ABM1RCCFS_flg] -> DTC_Info/3
  [VDDM_C1ABM1RCPass_flg] -> DTC_Info/2
  DTC_Info/1 -> VDDM_C1ABM1RCDTC_raw32/1  "VDDM_C1ABM1RCDTC_raw32"
  [task_time_s] -> Timer1/3
  [VPMM_PwrStaSW_enum] -> Equal2/1
  [VPMM_PwrStaSW_enum] -> Equal/1
  [VPMM_PowerSta_enum] -> Equal4/1
  [EDriveSysErr_VCUErr_flg] -> RC_EDriveSysErr_VCUErr_flg/1
  Constant4/1 -> Equal4/2
  Logical Operator8/1 -> Switch4/2
  Equal/1 -> Logical Operator2/2
  Constant28/1 -> Equal2/2
  Logical Operator5/1 -> Switch6/2
  Logical Operator6/1 -> Timer1/1
  [VDDM_C1ABM1RCChk_flg] -> Switch6/1
  Timer1/1 -> Equal3/1
  Equal3/1 -> SR_Latch1/1(set)
  Logical Operator1/1 -> Logical Operator2/3
  [task_time_s] -> Test Detection Criteria/2
  [VDDM_C1ABM1LCCFS_flg] -> Logical Operator4/1
  [VDDM_xxx_flg] -> SR_Latch1/2(reset)
  Switch/1 -> [EDriveSysErr_VCUErr_flg]
  Constant21/1 -> Switch/3
  [DTC_clear_request] -> Logical Operator8/2
  Constant16/1 -> Switch6/3
  Logical Operator2/1 -> Switch5/2
  Constant25/1 -> Switch4/3
  [No_CAN1_BUS_OFF] -> Logical Operator2/1
  Equal4/1 -> Logical Operator8/1
  Constant19/1 -> Equal3/2
  Constant26/1 -> Equal/2
  Constant40/1 -> Test Detection Criteria/3
  [VDDM_C1ABM1RCChk_flg] -> Switch5/1
  Logical Operator4/1 -> Logical Operator5/3
  Test Detection Criteria/1 -> [VDDM_C1ABM1RCDet_flg]  "VDDM_C1ABM1RCDet_flg"
  [VDDM_C1ABM1LCCFS_flg] -> Logical Operator1/1
  Constant18/1 -> Timer1/4
  Constant3/1 -> Switch/1
  [VDDM_C1ABM1RCCFS_flg] -> Switch/2
  Constant24/1 -> Switch4/1
  Switch4/1 -> [VDDM_C1ABM1RCCFSRls_flg]  "VDDM_C1ABM1RCCFSRls_flg"
  Switch6/1 -> Timer1/2, Logical Operator6/1
  Constant27/1 -> Switch5/3
  [No_CAN1_BUS_OFF] -> Logical Operator5/1
  SR_Latch1/1(latched) -> [VDDM_C1ABM1RCPass_flg]  "VDDM_C1ABM1RCPass_flg"
  Equal2/1 -> Logical Operator5/2
  DTC_clear_request/1 -> [DTC_clear_request]
  No_CAN1_BUS_OFF/1 -> [No_CAN1_BUS_OFF]
  VDDM_C1ABM1LCCFS_flg/1 -> [VDDM_C1ABM1LCCFS_flg]
  VPMM_PowerSta_enum/1 -> [VPMM_PowerSta_enum]
  VPMM_PwrStaSW_enum/1 -> [VPMM_PwrStaSW_enum]
  VDDM_C1ABM1RCChk_flg/1 -> [VDDM_C1ABM1RCChk_flg]
  task_time_s/1 -> [task_time_s]

== system ddm/DDM/DDM/PMM/Comm err/The CAN signal between VCU and ABM1 is incomplete ==
  note: Diagnostics and Fault Handling
  note: Test Pass Criteria
  note: Test Detection Criteria
  note: Release Condition During Failure Detection
  note: Fail Safe After Decision
  note: Release Condition After Failure Decision
  note: Fail Safe During Detection
  task_time_s : Inport
  VPMM_PowerSta_enum : Inport  Port=2
  VPMM_PwrStaSW_enum : Inport  Port=3
  VDDM_C1ABM1CSChk_flg : Inport  Port=4
  VDDM_C1ABM1LCCFS_flg : Inport  Port=5
  No_CAN1_BUS_OFF : Inport  Port=6
  DTC_clear_request : Inport  Port=7
  Constant15 : Constant  Value=KDDM_C1ABM1CSCFSSW_flg
  Constant16 : Constant  Value=TRUE
  Constant18 : Constant  Value=KDDM_C1ABM1CSPassTO_s
  Constant19 : Constant  Value=KDDM_C1ABM1CSPassTO_s
  Constant{2,21,25,27} (4 alike) : Constant  Value=FALSE
  Constant20 : Constant  Value=KDDM_C1ABM1CSDFSSW_flg
  Constant24 : Constant  Value=TRUE
  Constant26 : Constant  Value=ENUM_PWRSTASW_OFF
  Constant28 : Constant  Value=ENUM_PWRSTASW_OFF
  Constant3 : Constant  Value=TRUE
  Constant4 : Constant  Value=ENUM_POWERSTA_OFF
  Constant40 : Constant  Value=KDDM_C1ABM1CSDTC_cnt
  Constant41 : Constant  Value=KDDM_C1ABM1CSDetTO_s
  Constant46 : Constant  Value=KDDM_C1ABM1CSDetSW_flg
  Constant48 : Constant  Value=KDDM_C1ABM1CSDTC_cnt
  Constant5 : Constant  Value=KDDM_C1ABM1CSPassSW_flg
  DTC_Couter : hcu_lib/Basic_Blocks/DTC_Couter
  DTC_Info : hcu_lib/Basic_Blocks/DTC_Info
  Data Type Conversion1 : DataTypeConversion  OutDataTypeStr=uint8
  Equal : RelationalOperator  Operator=~=  OutDataTypeStr=boolean  RndMeth=Simplest
  Equal2 : RelationalOperator  Operator=~=  OutDataTypeStr=boolean  RndMeth=Simplest
  Equal3 : RelationalOperator  OutDataTypeStr=boolean  RndMeth=Simplest
  Equal4 : RelationalOperator  Operator===  OutDataTypeStr=boolean  RndMeth=Simplest
  Logical Operator{1,4,6..7} (4 alike) : Logic  Operator=NOT  AllPortsSameDT=off  OutDataTypeStr=boolean
  Logical Operator10 : Logic  Operator=OR  AllPortsSameDT=off  OutDataTypeStr=boolean
  Logical Operator12 : Logic  AllPortsSameDT=off  OutDataTypeStr=boolean
  Logical Operator15 : Logic  AllPortsSameDT=off  OutDataTypeStr=boolean
  Logical Operator18 : Logic  AllPortsSameDT=off  OutDataTypeStr=boolean
  Logical Operator19 : Logic  Inputs=3  AllPortsSameDT=off  OutDataTypeStr=boolean
  Logical Operator2 : Logic  Inputs=3  AllPortsSameDT=off  OutDataTypeStr=boolean
  Logical Operator3 : Logic  Operator=OR  Inputs=3  AllPortsSameDT=off  OutDataTypeStr=boolean
  Logical Operator5 : Logic  Inputs=3  AllPortsSameDT=off  OutDataTypeStr=boolean
  Logical Operator8 : Logic  Operator=OR  AllPortsSameDT=off  OutDataTypeStr=boolean
  Logical Operator9 : Logic  Operator=OR  AllPortsSameDT=off  OutDataTypeStr=boolean
  Relay : Relay  OnSwitchValue=ONE_INT  OffSwitchValue=ZERO_INT
  SR_Latch1 : Subsystem  mask(SR_Latch){}
      mask help: SR latch function.
  SR_Latch3 : hcu_lib/Basic_Blocks/SR_Latch
  SR_Latch4 : hcu_lib/Basic_Blocks/SR_Latch
  Switch{,1,4..6} (5 alike) : Switch  Criteria=u2 ~= 0
  Test Detection Criteria : hcu_lib/Basic_Blocks/Test Detection Criteria
  Timer1 : hcu_lib/Basic_Blocks/Timer
  VDDM_C1ABM1CSDTC_raw32 : Outport
  CS_EDriveSysErr_VCUErr_flg : Outport  Port=2
  wires:
  Logical Operator3/1 -> Logical Operator15/1
  Constant15/1 -> Logical Operator18/2
  DTC_Couter/1 -> SR_Latch4/1
  Logical Operator12/1 -> [VDDM_C1ABM1CSDFS_flg]  "VDDM_C1ABM1CSDFS_flg"
  Constant5/1 -> Logical Operator15/2
  Logical Operator7/1 -> Logical Operator19/3
  Data Type Conversion1/1 -> [VDDM_C1ABM1CSDTC_cnt]  "VDDM_C1ABM1CSDTC_cnt"
  [DTC_clear_request] -> Logical Operator10/2
  Logical Operator19/1 -> DTC_Couter/1
  [VDDM_C1ABM1CSCFSRls_flg] -> Logical Operator9/1
  SR_Latch3/1 -> Logical Operator12/2
  [VDDM_C1ABM1CSCFS_flg] -> Logical Operator10/1
  Constant46/1 -> Logical Operator19/2
  Constant20/1 -> Logical Operator12/1
  [VDDM_C1ABM1CSDet_flg] -> Logical Operator19/1
  DTC_Couter/2 -> Data Type Conversion1/1
  [VDDM_C1ABM1CSDTC_cnt] -> Relay/1
  SR_Latch4/1 -> Logical Operator18/1
  [DTC_clear_request] -> Logical Operator3/3
  Relay/1 -> SR_Latch3/1
  Logical Operator18/1 -> [VDDM_C1ABM1CSCFS_flg]  "VDDM_C1ABM1CSCFS_flg"
  [VDDM_C1ABM1CSPass_flg] -> Logical Operator3/1
  Logical Operator15/1 -> DTC_Couter/2
  Logical Operator10/1 -> SR_Latch3/2
  [DTC_clear_request] -> Logical Operator9/2
  [DTC_clear_request] -> Logical Operator7/1
  Logical Operator9/1 -> SR_Latch4/2
  [VDDM_C1ABM1CSCFSRls_flg] -> Logical Operator3/2
  Constant48/1 -> DTC_Couter/3
  Constant2/1 -> Switch1/1
  Switch5/1 -> Switch1/3, [VDDM_xxx_flg]
  Switch1/1 -> Test Detection Criteria/1
  [DTC_clear_request] -> Switch1/2
  [DTC_clear_request] -> DTC_Info/4
  Constant41/1 -> Test Detection Criteria/4
  [VDDM_C1ABM1CSDet_flg] -> DTC_Info/1
  [VDDM_C1ABM1CSPass_flg] -> DTC_Info/2
  [VDDM_C1ABM1CSCFS_flg] -> DTC_Info/3
  DTC_Info/1 -> VDDM_C1ABM1CSDTC_raw32/1  "VDDM_C1ABM1CSDTC_raw32"
  [task_time_s] -> Timer1/3
  [VPMM_PwrStaSW_enum] -> Equal2/1
  [VPMM_PwrStaSW_enum] -> Equal/1
  [VPMM_PowerSta_enum] -> Equal4/1
  [EDriveSysErr_VCUErr_flg] -> CS_EDriveSysErr_VCUErr_flg/1
  Constant3/1 -> Switch/1
  Constant19/1 -> Equal3/2
  Constant40/1 -> Test Detection Criteria/3
  Constant16/1 -> Switch6/3
  [VDDM_C1ABM1CSChk_flg] -> Switch5/1
  Logical Operator4/1 -> Logical Operator5/3
  Timer1/1 -> Equal3/1
  Constant26/1 -> Equal/2
  Equal4/1 -> Logical Operator8/1
  [No_CAN1_BUS_OFF] -> Logical Operator2/1
  Constant25/1 -> Switch4/3
  Logical Operator2/1 -> Switch5/2
  [No_CAN1_BUS_OFF] -> Logical Operator5/1
  Equal/1 -> Logical Operator2/2
  [DTC_clear_request] -> Logical Operator8/2
  Logical Operator6/1 -> Timer1/1
  Constant21/1 -> Switch/3
  Switch/1 -> [EDriveSysErr_VCUErr_flg]
  [VDDM_xxx_flg] -> SR_Latch1/2(reset)
  [VDDM_C1ABM1LCCFS_flg] -> Logical Operator4/1
  Logical Operator5/1 -> Switch6/2
  Logical Operator1/1 -> Logical Operator2/3
  [task_time_s] -> Test Detection Criteria/2
  Equal3/1 -> SR_Latch1/1(set)
  [VDDM_C1ABM1CSChk_flg] -> Switch6/1
  Constant28/1 -> Equal2/2
  Switch6/1 -> Timer1/2, Logical Operator6/1
  Switch4/1 -> [VDDM_C1ABM1CSCFSRls_flg]  "VDDM_C1ABM1CSCFSRls_flg"
  Constant27/1 -> Switch5/3
  Constant24/1 -> Switch4/1
  [VDDM_C1ABM1CSCFS_flg] -> Switch/2
  Logical Operator8/1 -> Switch4/2
  Constant18/1 -> Timer1/4
  [VDDM_C1ABM1LCCFS_flg] -> Logical Operator1/1
  Test Detection Criteria/1 -> [VDDM_C1ABM1CSDet_flg]  "VDDM_C1ABM1CSDet_flg"
  SR_Latch1/1(latched) -> [VDDM_C1ABM1CSPass_flg]  "VDDM_C1ABM1CSPass_flg"
  Equal2/1 -> Logical Operator5/2
  Constant4/1 -> Equal4/2
  No_CAN1_BUS_OFF/1 -> [No_CAN1_BUS_OFF]
  DTC_clear_request/1 -> [DTC_clear_request]
  task_time_s/1 -> [task_time_s]
  VDDM_C1ABM1CSChk_flg/1 -> [VDDM_C1ABM1CSChk_flg]
  VPMM_PwrStaSW_enum/1 -> [VPMM_PwrStaSW_enum]
  VPMM_PowerSta_enum/1 -> [VPMM_PowerSta_enum]
  VDDM_C1ABM1LCCFS_flg/1 -> [VDDM_C1ABM1LCCFS_flg]

== system ddm/DDM/DDM/PMM/Comm err/The CAN signal between VCU and BMS1 is discontinuous ==
  note: Diagnostics and Fault Handling
  note: Test Detection Criteria
  note: Fail Safe During Detection
  note: Fail Safe After Decision
  note: Release Condition During Failure Detection
  note: Release Condition After Failure Decision
  note: Test Pass Criteria
  task_time_s : Inport
  VPMM_PowerSta_enum : Inport  Port=2
  VPMM_PwrStaSW_enum : Inport  Port=3
  VDDM_C3BMS1RCChk_flg : Inport  Port=4
  VDDM_C3BMS1LCCFS_flg : Inport  Port=5
  No_CAN3_BUS_OFF : Inport  Port=6
  DTC_clear_request : Inport  Port=7
  Constant15 : Constant  Value=KDDM_C3BMS1RCCFSSW_flg
  Constant{3,16,22,24} (4 alike) : Constant  Value=TRUE
  Constant18 : Constant  Value=KDDM_C3BMS1RCPassTO_s
  Constant19 : Constant  Value=KDDM_C3BMS1RCPassTO_s
  Constant{2,21,23,25,27} (5 alike) : Constant  Value=FALSE
  Constant20 : Constant  Value=KDDM_C3BMS1RCDFSSW_flg
  Constant26 : Constant  Value=ENUM_PWRSTASW_OFF
  Constant28 : Constant  Value=ENUM_PWRSTASW_OFF
  Constant4 : Constant  Value=ENUM_POWERSTA_OFF
  Constant40 : Constant  Value=KDDM_C3BMS1RCDTC_cnt
  Constant41 : Constant  Value=KDDM_C3BMS1RCDetTO_s
  Constant46 : Constant  Value=KDDM_C3BMS1RCDetSW_flg
  Constant48 : Constant  Value=KDDM_C3BMS1RCDTC_cnt
  Constant5 : Constant  Value=KDDM_C3BMS1RCPassSW_flg
  DTC_Couter : hcu_lib/Basic_Blocks/DTC_Couter
  DTC_Info : hcu_lib/Basic_Blocks/DTC_Info
  Data Type Conversion1 : DataTypeConversion  OutDataTypeStr=uint8
  Demux : Demux  Commented=on  Outputs=5
  Equal : RelationalOperator  Operator=~=  OutDataTypeStr=boolean  RndMeth=Simplest
  Equal2 : RelationalOperator  Operator=~=  OutDataTypeStr=boolean  RndMeth=Simplest
  Equal3 : RelationalOperator  OutDataTypeStr=boolean  RndMeth=Simplest
  Equal4 : RelationalOperator  Operator===  OutDataTypeStr=boolean  RndMeth=Simplest
  From19 : From  Commented=on  GotoTag=VDDM_C3BMS1RCDFS_flg
  Goto19 : Goto  Commented=on  GotoTag=VDDM_EDriveSysErrVCUErr_flg
  Logical Operator{1,4,6,9} (4 alike) : Logic  Operator=NOT  AllPortsSameDT=off  OutDataTypeStr=boolean
  Logical Operator12 : Logic  AllPortsSameDT=off  OutDataTypeStr=boolean
  Logical Operator15 : Logic  AllPortsSameDT=off  OutDataTypeStr=boolean
  Logical Operator18 : Logic  AllPortsSameDT=off  OutDataTypeStr=boolean
  Logical Operator19 : Logic  Inputs=3  AllPortsSameDT=off  OutDataTypeStr=boolean
  Logical Operator2 : Logic  Inputs=3  AllPortsSameDT=off  OutDataTypeStr=boolean
  Logical Operator21 : Logic  Operator=OR  Inputs=3  AllPortsSameDT=off  OutDataTypeStr=boolean
  Logical Operator3 : Logic  Operator=OR  Inputs=3  AllPortsSameDT=off  OutDataTypeStr=boolean
  Logical Operator5 : Logic  Inputs=3  AllPortsSameDT=off  OutDataTypeStr=boolean
  Logical Operator7 : Logic  Operator=OR  AllPortsSameDT=off  OutDataTypeStr=boolean
  Logical Operator8 : Logic  Operator=OR  AllPortsSameDT=off  OutDataTypeStr=boolean
  Relay : Relay  OnSwitchValue=ONE_INT  OffSwitchValue=ZERO_INT
  SR_Latch1 : Subsystem  mask(SR_Latch){}
      mask help: SR latch function.
  SR_Latch3 : hcu_lib/Basic_Blocks/SR_Latch
  SR_Latch4 : hcu_lib/Basic_Blocks/SR_Latch
  Switch{,1,4..7} (6 alike) : Switch  Criteria=u2 ~= 0
  Switch3 : Switch  Commented=on  Criteria=u2 ~= 0
  Test Detection Criteria1 : hcu_lib/Basic_Blocks/Test Detection Criteria
  Timer1 : hcu_lib/Basic_Blocks/Timer
  Unit Delay3 : UnitDelay  Commented=on  SampleTime=-1  HasFrameUpgradeWarning=on
  VDDM_C3BMS1RCDTC_raw32 : Outport
  wires:
  [VDDM_C3BMS1RCDTC_cnt] -> Relay/1
  [DTC_clear_request] -> Logical Operator9/1
  Logical Operator19/1 -> DTC_Couter/1
  Logical Operator21/1 -> SR_Latch3/2
  Logical Operator7/1 -> SR_Latch4/2
  [DTC_clear_request] -> Logical Operator7/2
  Constant48/1 -> DTC_Couter/3
  [VDDM_C3BMS1RCCFS_flg] -> Logical Operator21/2
  Logical Operator9/1 -> Logical Operator19/3
  DTC_Couter/2 -> Data Type Conversion1/1
  Logical Operator3/1 -> Logical Operator15/1
  Data Type Conversion1/1 -> [VDDM_C3BMS1RCDTC_cnt]  "VDDM_C3BMS1RCDTC_cnt"
  Logical Operator18/1 -> [VDDM_C3BMS1RCCFS_flg]  "VDDM_C3BMS1RCCFS_flg"
  [VDDM_C3BMS1RCDFSRls_flg] -> Logical Operator21/1
  SR_Latch3/1 -> Logical Operator12/2
  [VDDM_C3BMS1RCCFSRls_flg] -> Logical Operator3/2
  Relay/1 -> SR_Latch3/1
  Constant5/1 -> Logical Operator15/2
  Logical Operator12/1 -> [VDDM_C3BMS1RCDFS_flg]  "VDDM_C3BMS1RCDFS_flg"
  DTC_Couter/1 -> SR_Latch4/1
  SR_Latch4/1 -> Logical Operator18/1
  [VDDM_C3BMS1RCPass_flg] -> Logical Operator3/1
  [DTC_clear_request] -> Logical Operator3/3
  [VDDM_C3BMS1RCDet_flg] -> Logical Operator19/1
  Constant46/1 -> Logical Operator19/2
  Constant15/1 -> Logical Operator18/2
  Constant20/1 -> Logical Operator12/1
  [VDDM_C3BMS1RCCFSRls_flg] -> Logical Operator7/1
  Logical Operator15/1 -> DTC_Couter/2
  [DTC_clear_request] -> Logical Operator21/3
  Constant2/1 -> Switch1/1
  Switch5/1 -> Switch1/3, [VDDM_xxx_flg]
  Switch1/1 -> Test Detection Criteria1/1
  [DTC_clear_request] -> Switch1/2
  [DTC_clear_request] -> DTC_Info/4
  Constant41/1 -> Test Detection Criteria1/4
  [VDDM_C3BMS1RCDet_flg] -> DTC_Info/1
  DTC_Info/1 -> VDDM_C3BMS1RCDTC_raw32/1  "VDDM_C3BMS1RCDTC_raw32"
  [VDDM_C3BMS1RCCFS_flg] -> DTC_Info/3
  [VDDM_C3BMS1RCPass_flg] -> DTC_Info/2
  [task_time_s] -> Timer1/3
  [VPMM_PwrStaSW_enum] -> Equal2/1
  [VPMM_PwrStaSW_enum] -> Equal/1
  [VPMM_PowerSta_enum] -> Equal4/1
  [VDDM_C3BMS1RCCFS_flg] -> Switch/2
  Constant3/1 -> Switch/1
  Switch6/1 -> Timer1/2, Logical Operator6/1
  Equal2/1 -> Logical Operator5/2
  Test Detection Criteria1/1 -> [VDDM_C3BMS1RCDet_flg]  "VDDM_C3BMS1RCDet_flg"
  Constant40/1 -> Test Detection Criteria1/3
  [task_time_s] -> Test Detection Criteria1/2
  [VDDM_C3BMS1RCChk_flg] -> Switch5/1
  Constant26/1 -> Equal/2
  Constant19/1 -> Equal3/2
  Logical Operator2/1 -> Switch5/2
  Equal/1 -> Logical Operator2/2
  Switch7/1 -> [VDDM_C3BMS1RCDFSRls_flg]  "VDDM_C3BMS1RCDFSRls_flg"
  [VDDM_xxx_flg] -> SR_Latch1/2(reset)
  [VDDM_C3BMS1RCChk_flg] -> Switch6/1
  Constant25/1 -> Switch4/3
  Constant21/1 -> Switch/3
  Constant23/1 -> Switch7/3
  [DTC_clear_request] -> Logical Operator8/2
  From19/1 -> Switch3/2
  Logical Operator8/1 -> Switch4/2
  Constant27/1 -> Switch5/3
  Constant16/1 -> Switch6/3
  [No_CAN3_BUS_OFF] -> Logical Operator2/1
  Constant28/1 -> Equal2/2
  SR_Latch1/1(latched) -> [VDDM_C3BMS1RCPass_flg]  "VDDM_C3BMS1RCPass_flg"
  Switch4/1 -> [VDDM_C3BMS1RCCFSRls_flg]  "VDDM_C3BMS1RCCFSRls_flg"
  Equal4/1 -> Logical Operator8/1
  [VDDM_C3BMS1RCPass_flg] -> Switch7/2
  Constant24/1 -> Switch4/1
  Logical Operator6/1 -> Timer1/1
  Switch/1 -> Goto19/1
  Timer1/1 -> Equal3/1
  Constant4/1 -> Equal4/2
  Constant22/1 -> Switch7/1
  Constant18/1 -> Timer1/4
  Equal3/1 -> SR_Latch1/1(set)
  Switch3/1 -> Demux/1
  Logical Operator4/1 -> Logical Operator5/3
  Logical Operator1/1 -> Logical Operator2/3
  Demux/1 -> Unit Delay3/1
  [No_CAN3_BUS_OFF] -> Logical Operator5/1
  Logical Operator5/1 -> Switch6/2
  [VDDM_C3BMS1LCCFS_flg] -> Logical Operator1/1
  [VDDM_C3BMS1LCCFS_flg] -> Logical Operator4/1
  DTC_clear_request/1 -> [DTC_clear_request]
  No_CAN3_BUS_OFF/1 -> [No_CAN3_BUS_OFF]
  VDDM_C3BMS1LCCFS_flg/1 -> [VDDM_C3BMS1LCCFS_flg]
  task_time_s/1 -> [task_time_s]
  VDDM_C3BMS1RCChk_flg/1 -> [VDDM_C3BMS1RCChk_flg]
  VPMM_PwrStaSW_enum/1 -> [VPMM_PwrStaSW_enum]
  VPMM_PowerSta_enum/1 -> [VPMM_PowerSta_enum]
